simulink model "baseline1"  (R2022b)
settings: Solver=ode4  StartTime=0.0  StopTime=200  FixedStep=1e-3  RelTol=1e-3
undefined symbols (not defined in the file or in its folder): A_do, B_do, c_uf, do_w, f_b, f_max, f_min, F_TOT_MAX, Fz_min, g, G_do, Gamma_mix, Ixx, Iyy, Izz, K_eta, K_omega, K_w, Ka1, Ka2, Ka3, Kgamma, Knu, Kp1, Kp2, Kp3, L, l_axis, l_gain, m, m_p, n_state_axis, p2_bias_acc, p2_h3_s0, p2_ic_do, p2_ic_eso, p2_ic_pos, p2_ic_vel, p2_nd_pos, p2_prm, p2_prm_h3, p2_prm_m3, p2_prm_n6, p2_prm_w, p2_seed_acc, p2_seed_gyro, p2_seed_pos, p2_tau_m, p2_trim_do, p2_trim_eso, p2_trim_ff_v, p2_Ts_att, p2_Ts_pos, p2_var_acc, p2_var_gyro, p2_var_pos, payload_amp, payload_inj_on, payload_K_ratio, payload_model ... (+18)
(part 3 of 3)

== matlab function baseline1/Attitude_Reference/Thrust_AttRef_16 ==
  data: F input; f output; eta input; psi_d input; Fz_min input; eta_d output; F_TOT_MAX input
function [f, eta_d] = thrust_attitude_ref(F, eta, psi_d, Fz_min, F_TOT_MAX)
%#codegen
% --- Khai bao kich thuoc output (de Simulink suy dung kich thuoc tin hieu) ---
f = 0; eta_d = zeros(3,1);
% Pt. (16) Guo 2020 + 2 gioi han an toan chuan autopilot [MOI]:
%  (a) kep goc nghieng lenh |phi_d|,|theta_d| <= 30 deg
%      -> nhat quan Assumption 4 (bay goc nho)
%  (b) kep tong luc day lenh f trong [0, 21.6] N (= 0.9*4*f_max, f_max = 6 N)
% Neu khong kep: khi Fz cham day Fz_min, atan2 cho goc lenh ~90 deg ->
% UAV lat -> mat luc nang thang dung -> phan ky. Thi nghiem that cua bai
% bao cat canh + bay toi diem dau quy dao truoc nen khong gap tinh huong nay.
TILT_MAX  = 30*pi/180;   % [MOI]
% F_TOT_MAX: input since GD2b (workspace variable F_TOT_MAX). v1 default 21.6
% (= 0.9*4*f_max, f_max = 6 N; init_MOBADC_params), the same double as the old
% literal. Plant P2: 0.9 x plant max = 27.603 N (PLANT_P2_SPEC sec 2.1).
Fx = F(1); Fy = F(2); Fz = max(F(3), Fz_min);
phi = eta(1); theta = eta(2); psi = eta(3);
cpsi = cos(psi); spsi = sin(psi);
theta_d = atan2(Fx*cpsi + Fy*spsi, Fz);
phi_d   = atan2(cos(theta_d)*(Fx*spsi - Fy*cpsi), Fz);
theta_d = min(max(theta_d, -TILT_MAX), TILT_MAX);
phi_d   = min(max(phi_d,   -TILT_MAX), TILT_MAX);
cc = max(cos(theta)*cos(phi), 0.5);    % f theo dong dau (16), goc thuc te
f  = min(max(Fz/cc, 0), F_TOT_MAX);
eta_d = [phi_d; theta_d; psi_d];
end

== matlab function baseline1/Rotational_Control/Att_Ctrl_18 ==
  data: eta_d input; tau_cmd output; eta input; omega input; dltau_hat input; K_eta input; K_omega input
function tau_cmd = attitude_controller(eta_d, eta, omega, dltau_hat, K_eta, K_omega)
%#codegen
% --- Khai bao kich thuoc output (de Simulink suy dung kich thuoc tin hieu) ---
tau_cmd = zeros(3,1);
% Luat dieu khien vong tu the, pt. (17)-(18) Guo 2020:
%   e_eta = eta_d - eta                                               (17)
%   tau_d = K_eta*e_eta - K_omega*omega - dltau_hat                   (18)
% omega la BODY rates (Remark 3: omega_d = 0). PID mode: dltau_hat = 0.
e_eta   = eta_d - eta;
tau_cmd = K_eta*e_eta - K_omega*omega - dltau_hat;
end

== matlab function baseline1/Motor_Allocation/Alloc_2_3 ==
  data: f_cmd input; f_act output; tau_cmd input; Gamma_mix input; f_min input; f_max input; c_uf input; f_b input; u_b input; tau_act output; f_i output; u_i output
function [f_act, tau_act, f_i, u_i] = motor_allocation(f_cmd, tau_cmd, Gamma_mix, f_min, f_max, c_uf, f_b, u_b)
%#codegen
% --- Khai bao kich thuoc output (de Simulink suy dung kich thuoc tin hieu) ---
f_act = 0; tau_act = zeros(3,1); f_i = zeros(4,1); u_i = zeros(4,1);
% Pt. (2) bai bao + bao hoa motor + kep moment lenh [MOI]:
% |tau_i| <= 0.5 N.m - dung dai lenh moment Fig. 11(b) cua bai bao.
% Kep tau TRUOC khi phan bo de giu quy luc cho moment, tranh ca 4 motor
% ket tran -> tau_act = 0 (mat dieu khien tu the).
TAU_MAX = 0.5;   % N.m [MOI - khop Fig. 11(b)]
tau_c   = min(max(tau_cmd, -TAU_MAX), TAU_MAX);
wrench  = [f_cmd; tau_c(1); tau_c(2); tau_c(3)];
f_i_raw = Gamma_mix \ wrench;                    % phan bo nguoc (2)
f_i     = min(max(f_i_raw, f_min), f_max);       % bao hoa tung motor
wrench_act = Gamma_mix * f_i;                    % tai hop luc/moment thuc
f_act   = wrench_act(1);
tau_act = wrench_act(2:4);
u_i = c_uf*sqrt(max(f_i - f_b, 0)) - u_b;        % pt. (3), chi de log
end

== matlab function baseline1/UAV_Plant/Force_4b ==
  data: f_act input; F_act output; eta input
function F_act = force_from_attitude(f_act, eta)
%#codegen
% --- Khai bao kich thuoc output (de Simulink suy dung kich thuoc tin hieu) ---
F_act = zeros(3,1);
% Pt. (4b) Guo 2020 - luc thuc te len khoi tam tu tong luc day f va
% GOC THUC TE eta (mat xich ghep vong tu the vao vong vi tri):
%   F = f*[c_psi*s_theta*c_phi + s_psi*s_phi;
%          s_psi*s_theta*c_phi - s_phi*c_psi;
%          c_theta*c_phi]
phi = eta(1); theta = eta(2); psi = eta(3);
cphi = cos(phi); sphi = sin(phi);
cth  = cos(theta); sth = sin(theta);
cpsi = cos(psi); spsi = sin(psi);
F_act = f_act*[cpsi*sth*cphi + spsi*sphi;
               spsi*sth*cphi - sphi*cpsi;
               cth*cphi];
end
